simulink model "gm_HDLModulatorFull_vs"  (R2024a)
settings: Solver=FixedStepDiscrete  StartTime=0.0  StopTime=stopTime  RelTol=1e-3
values from neighbouring files (symbols this model uses):
  dataSymbols = [ ... (first row only)    [testModulatorFull.m]
undefined symbols (not defined in the file or in its folder): clk, clk_enable, fPHY, fs, interpolatorDelay, interpolatorFilter, N, numDataCarriers, oversamplingFactor, reset_x
libraries: hdlmdlgenlib x54, hdlsllib x21, dspsrcs4 x4, commdigbbndam3 x4, simulink x3, dspsigops x2, whdlutilities x1, dsphdlsigops2 x1, dsphdlfiltering2 x1, whdlmod x1, vivadosimlib x1, HDL_ieee_8021513 x1
settings Model: Creator=cotti  LastModifiedBy=cotti
settings OptimizationCC: BlockReduction=off  ConditionallyExecuteInputs=off  DefaultParameterBehavior=Inlined  InheritOutputTypeSmallerThanSingle=on
settings DebuggingCC: AlgebraicLoopMsg=error  ArtificialAlgebraicLoopMsg=error  InheritedTsInSrcMsg=none  SingleTaskRateTransMsg=error  UnconnectedInputMsg=warning  UnconnectedOutputMsg=warning  UnconnectedLineMsg=warning
settings HardwareCC: ProdBitPerPointer=32  ProdBitPerSizeT=32  ProdBitPerPtrDiffT=32  ProdLargestAtomicFloat=None  ProdIntDivRoundTo=Undefined  ProdEndianess=Unspecified  ProdWordSize=32  ProdHWDeviceType=ASIC/FPGA->ASIC/FPGA  TargetBitPerLong=64  TargetBitPerPointer=64  TargetBitPerSizeT=64  TargetBitPerPtrDiffT=64  TargetLongLongMode=on  TargetIntDivRoundTo=Zero  TargetEndianess=LittleEndian  TargetWordSize=64  TargetHWDeviceType=Custom Processor->MATLAB Host Computer  ProdEqTarget=off

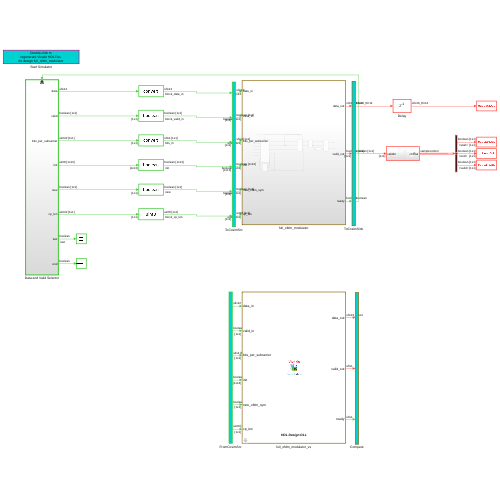
[thumbnail: Simulink's stored preview of the top-level diagram]
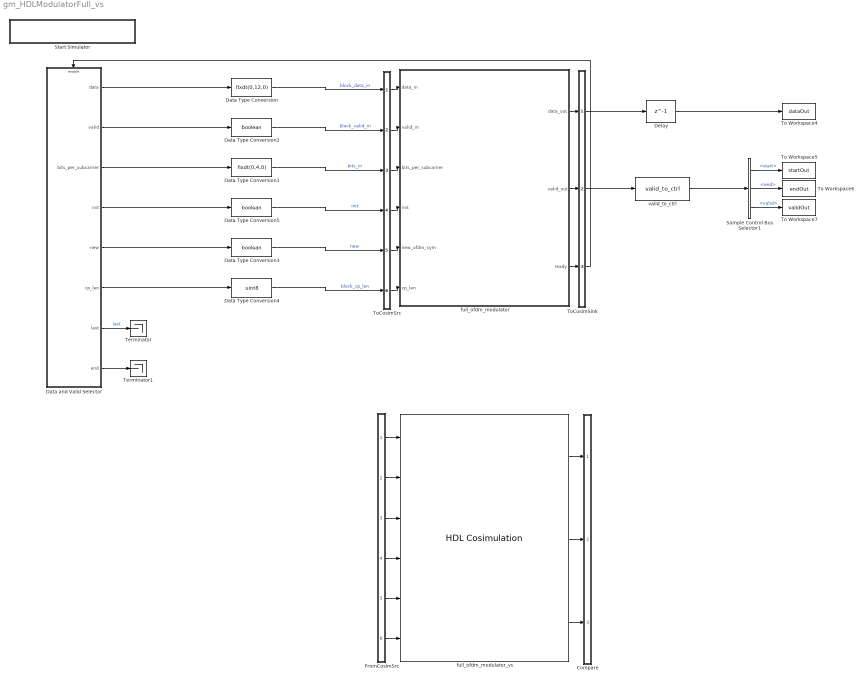
== system gm_HDLModulatorFull_vs ==
  Compare : Subsystem
      mask Display: disp('')
  Data Type Conversion : DataTypeConversion  OutDataTypeStr=fixdt(0,12,0)  SaturateOnIntegerOverflow=off  RndMeth=Floor  LockScale=on
  Data Type Conversion1 : DataTypeConversion  OutDataTypeStr=fixdt(0,4,0)  SaturateOnIntegerOverflow=off  RndMeth=Floor  LockScale=on
  Data Type Conversion2 : DataTypeConversion  OutDataTypeStr=boolean  SaturateOnIntegerOverflow=off  RndMeth=Floor  LockScale=on
  Data Type Conversion3 : DataTypeConversion  OutDataTypeStr=boolean  SaturateOnIntegerOverflow=off  RndMeth=Floor  LockScale=on
  Data Type Conversion4 : DataTypeConversion  OutDataTypeStr=uint8  SaturateOnIntegerOverflow=off  RndMeth=Floor  LockScale=on
  Data Type Conversion5 : DataTypeConversion  OutDataTypeStr=boolean  SaturateOnIntegerOverflow=off  RndMeth=Floor  LockScale=on
  Data and Valid Selector : Subsystem  TreatAsAtomicUnit=on
  Delay : Delay  DelayLength=1  InitialCondition=0  UseCircularBuffer=on
  FromCosimSrc : Subsystem
      mask Display: disp('')
  Sample Control Bus Selector1 : whdlutilities/Sample Control Bus Selector  OutputSignals=start,end,valid
  Start Simulator : Subsystem
      settings: OpenFcn=|
      | cosimDirName = pwd;
      | cd 'hdl_prj/hdlsrc/HDLModulatorFull';
      | [s,r] = system('vivado -mode batch -source gm_HDLModulatorFull_vs.tcl','-echo');
      | cd (cosimDirName);
      | clear cosimDirName;
      | if s
      |    error('Failed to create Vivado HDL design DLL using script gm_HDLModulatorFull_vs.tcl.');
      | end
      mask Display: disp('Double-click to\nregenerate Vivado HDL DLL\nfor design full_ofdm_modulator')
  Terminator : Terminator
  Terminator1 : Terminator
  To Workspace4 : ToWorkspace  VariableName=dataOut  SampleTime=1/fs
      settings: Save2DSignal=2-D array (concatenate along first dimension)
  To Workspace5 : ToWorkspace  VariableName=startOut  SampleTime=1/fs
      settings: Save2DSignal=2-D array (concatenate along first dimension)
  To Workspace6 : ToWorkspace  VariableName=endOut  SampleTime=1/fs
      settings: Save2DSignal=2-D array (concatenate along first dimension)
  To Workspace7 : ToWorkspace  VariableName=validOut  SampleTime=1/fs
      settings: Save2DSignal=2-D array (concatenate along first dimension)
  ToCosimSink : Subsystem
      mask Display: disp('')
  ToCosimSrc : Subsystem
      mask Display: disp('')
  full_ofdm_modulator : Subsystem
  full_ofdm_modulator_vs : vivadosimlib/HDL Cosimulation  PortPaths=/full_ofdm_modulator/data_in;/full_ofdm_modulator/valid_in;/full_ofdm_modulator/bits_per_subcarrier;/full_ofdm_modulator/init;/full_ofdm_modulator/new_ofdm_sym;/full_ofdm_modulator/cp_len;/full_ofdm_modulator/data_out;/full_ofdm_modulator/valid_out;/full_ofdm_modulator/ready  PortModes=[1 1 1 1 1 1 2 2 2 ]  PortTimes=[-1 -1 -1 -1 -1 -1 1.0000000000000000209225608301284726753266340892878361046314239502e-08 1.0000000000000000209225608301284726753266340892878361046314239502e-08 2.0000000000000000418451216602569453506532681785756722092628479004e-08 ]  PortSigns=[-1 -1 -1 -1 -1 -1 1 0 0 ]  PortFracLengths=[0,0,0,0,0,0,14,0,0]  PortWordLengths=[-1,-1,-1,-1,-1,-1,16,1,1]  PortHDLWordSizes=[12,1,4,1,1,8,16,1,1]  CommLocal=on  CommSharedMemory=on  CommPortNumber=4449  CommShowInfo=on  ClockPaths=clk;clk_enable;reset_x;  ClockModes=[2 4 3]  ClockTimes=[1e-08 3.7e-08 2.7e-08]  TclPostSimCommand="puts \"done\""  TimingMode=ns  TimingScaleFactor=1000000000  idxCellArray={'UNUSED_VAR'}  CosimBypass=Full Simulation  AllowDirectFeedthrough=on  ProductName=EDA Simulator Link VS  RunAutoTimescale=off  HdlClocks=0  PreRunTime=40  PreRunTimeUnit=ns
  valid_to_ctrl : HDL_ieee_8021513/valid_to_ctrl  SystemSampleTime=-1  VariantActivationTime=update diagram  AllowFlexibleInterface=on  Latency=0  AutoFrameSizeCalculation=off
      settings: SourceProductName=HDL IEEE 8021513
  wires:
  Sample Control Bus Selector1/3 -> To Workspace7/1  "<valid>"
  valid_to_ctrl/1 -> Sample Control Bus Selector1/1
  Sample Control Bus Selector1/1 -> To Workspace5/1  "<start>"
  Sample Control Bus Selector1/2 -> To Workspace6/1  "<end>"
  Data and Valid Selector/8(end) -> Terminator1/1
  Data and Valid Selector/6(cp_len) -> Data Type Conversion4/1
  Data and Valid Selector/4(init) -> Data Type Conversion5/1
  Data and Valid Selector/2(valid) -> Data Type Conversion2/1
  Data and Valid Selector/1(data) -> Data Type Conversion/1
  Data and Valid Selector/3(bits_per_subcarrier) -> Data Type Conversion1/1
  Data and Valid Selector/5(new) -> Data Type Conversion3/1
  Data and Valid Selector/7(last) -> Terminator/1  "last"
  Delay/1 -> To Workspace4/1
  ToCosimSrc/1(out1) -> full_ofdm_modulator/1(data_in)
  ToCosimSrc/2(out2) -> full_ofdm_modulator/2(valid_in)
  ToCosimSrc/3(out3) -> full_ofdm_modulator/3(bits_per_subcarrier)
  ToCosimSrc/4(out4) -> full_ofdm_modulator/4(init)
  ToCosimSrc/5(out5) -> full_ofdm_modulator/5(new_ofdm_sym)
  ToCosimSrc/6(out6) -> full_ofdm_modulator/6(cp_len)
  full_ofdm_modulator/1(data_out) -> ToCosimSink/1(in1)
  full_ofdm_modulator/2(valid_out) -> ToCosimSink/2(in2)
  full_ofdm_modulator/3(ready) -> ToCosimSink/3(in3)
  Data Type Conversion/1 -> ToCosimSrc/1(in1)  "block_data_in"
  Data Type Conversion2/1 -> ToCosimSrc/2(in2)  "block_valid_in"
  Data Type Conversion1/1 -> ToCosimSrc/3(in3)  "bits_in"
  Data Type Conversion5/1 -> ToCosimSrc/4(in4)  "init"
  Data Type Conversion3/1 -> ToCosimSrc/5(in5)  "new"
  Data Type Conversion4/1 -> ToCosimSrc/6(in6)  "block_cp_len"
  ToCosimSink/1(out1) -> Delay/1
  ToCosimSink/2(out2) -> valid_to_ctrl/1
  ToCosimSink/3(out3) -> Data and Valid Selector/Enable
  FromCosimSrc/1(out1) -> full_ofdm_modulator_vs/1
  FromCosimSrc/2(out2) -> full_ofdm_modulator_vs/2
  FromCosimSrc/3(out3) -> full_ofdm_modulator_vs/3
  FromCosimSrc/4(out4) -> full_ofdm_modulator_vs/4
  FromCosimSrc/5(out5) -> full_ofdm_modulator_vs/5
  FromCosimSrc/6(out6) -> full_ofdm_modulator_vs/6
  full_ofdm_modulator_vs/1 -> Compare/1(in1)
  full_ofdm_modulator_vs/2 -> Compare/2(in2)
  full_ofdm_modulator_vs/3 -> Compare/3(in3)

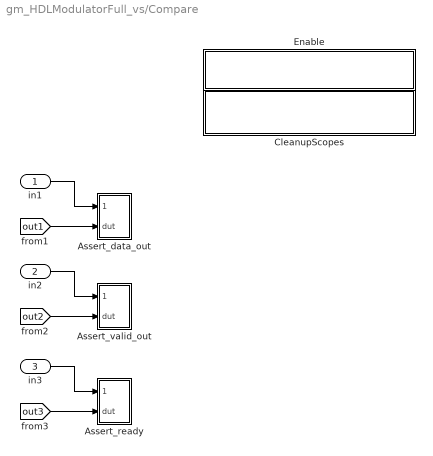
== system gm_HDLModulatorFull_vs/Compare ==
  in1 : Inport
  in2 : Inport  Port=2
  in3 : Inport  Port=3
  Assert_data_out : Subsystem
      settings: LibrarySourceBlock=hdlmdlgenlib/AssertEq
  Assert_ready : Subsystem
      settings: LibrarySourceBlock=hdlmdlgenlib/AssertEq
  Assert_valid_out : Subsystem
      settings: LibrarySourceBlock=hdlmdlgenlib/AssertEq
  CleanupScopes : Subsystem
      settings: OpenFcn=|
      | blkName = gcb; %self block
      | idx = regexp(blkName, '/CleanupScopes$', 'once');
      | blkParent = blkName(1:idx-1);
      | blks=find_system(blkParent, 'LookUnderMasks', 'all','blocktype', 'Scope');
      | for itr = 1:length(blks)
      | 	 hScopeCfg = get_param(blks{itr},'ScopeConfiguration');
      | 	 hScopeCfg.Visible = ~ hScopeCfg.Visible;
      | end
      | drawnow;
      mask Display: fprintf(message('hdlcoder:cosim:vnl_dblclick').getString());
  Enable : Subsystem
      settings: OpenFcn=|
      | blkName = gcb;
      | idx = regexp(blkName, '/Enable$', 'once');
      | blkParent = blkName(1:idx-1);
      | blks=find_system(blkParent, 'LookUnderMasks', 'all','blocktype', 'Assertion');
      | e = get_param(blks{1}, 'Enabled');
      | if strcmp(e, 'on'), f= 'off';, else, f = 'on';, end
      | for ii=1:length(blks), set_param(blks{ii}, 'Enabled', f);, end
      | set_param(gcb, 'MaskDisplay',['fprintf(message(''hdlcoder:cosim:vnl_dblclick_assertions'',','''',upper(e),'''',').getString())']);
      mask Display: fprintf(message('hdlcoder:cosim:vnl_dblclick_assertions','OFF').getString());
  wires:
  in3/1 -> Assert_ready/1(cosim)
  [out2] -> Assert_valid_out/2(dut)
  [out3] -> Assert_ready/2(dut)
  in2/1 -> Assert_valid_out/1(cosim)
  [out1] -> Assert_data_out/2(dut)
  in1/1 -> Assert_data_out/1(cosim)

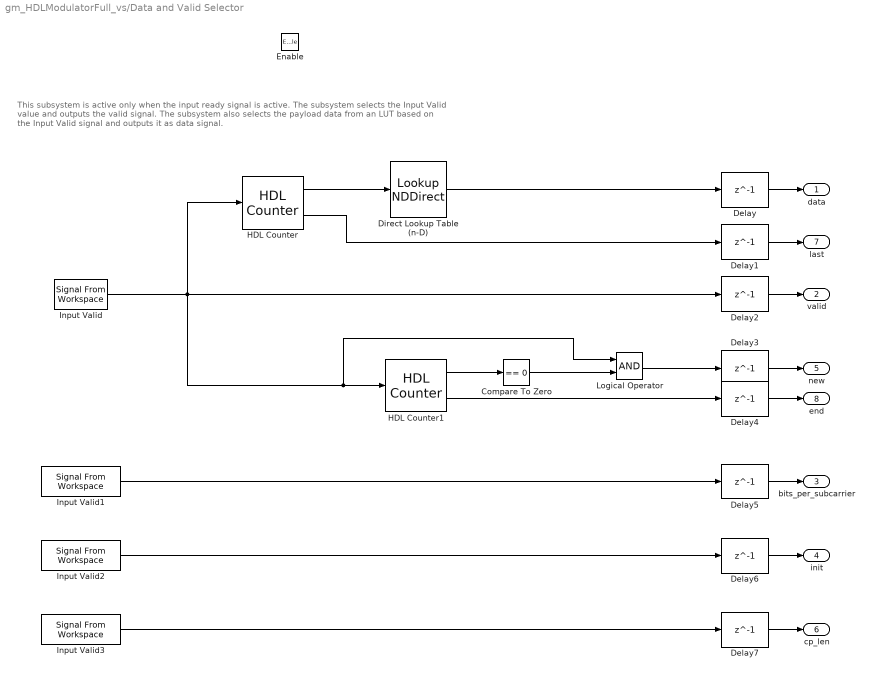
== system gm_HDLModulatorFull_vs/Data and Valid Selector ==
  note: This subsystem is active only when the input ready signal is active. The subsystem selects the Input Valid value and outputs the valid signal.
      | The subsystem also selects the payload data from an LUT based on the Input Valid signal and outputs it as data signal.
  Enable : EnablePort
  Compare To Zero : hdlsllib/Logic and Bit Operations/Compare To Zero  relop===  OutDataTypeStr=boolean
  Delay{,1..7} (8 alike) : Delay  DelayLength=1  InitialCondition=0  UseCircularBuffer=on
  Direct Lookup Table (n-D) : LookupNDDirect  NumberOfTableDimensions=1  Table=dataSymbols  DiagnosticForOutOfRangeInput=Error  TableDataTypeStr=fixdt(0,12,0)
  HDL Counter : hdlsllib/Sources/HDL Counter  CountType=Count limited  CountInit=0  CountStep=1  CountMax=length(dataSymbols) -1  CountFromType=Initial value  CountFrom=0  CountResetPort=off  CountLoadPort=off  CountEnbPort=on  CountDirPort=off  CountHitOutputPort=on  CountDataType=Unsigned  CountWordLen=nextpow2(length(dataSymbols))  CountFracLen=0  CountSampTime=1
  HDL Counter1 : hdlsllib/Sources/HDL Counter  CountType=Count limited  CountInit=0  CountStep=1  CountMax=numDataCarriers-1  CountFromType=Initial value  CountFrom=0  CountResetPort=off  CountLoadPort=off  CountEnbPort=on  CountDirPort=off  CountHitOutputPort=on  CountDataType=Unsigned  CountWordLen=nextpow2(numDataCarriers)  CountFracLen=0  CountSampTime=1
  Input Valid : dspsrcs4/Signal From Workspace  X=validIn  Ts=1/fPHY  nsamps=1  OutputAfterFinalValue=Setting to zero  ignoreOrWarnInputAndFrameLengths=off  OutputFrames=off
  Input Valid1 : dspsrcs4/Signal From Workspace  X=bitsPerSubcarrier  Ts=1/fPHY  nsamps=1  OutputAfterFinalValue=Setting to zero  ignoreOrWarnInputAndFrameLengths=off  OutputFrames=off
  Input Valid2 : dspsrcs4/Signal From Workspace  X=init  Ts=1/fPHY  nsamps=1  OutputAfterFinalValue=Setting to zero  ignoreOrWarnInputAndFrameLengths=off  OutputFrames=off
  Input Valid3 : dspsrcs4/Signal From Workspace  X=cpLen  Ts=1/fPHY  nsamps=1  OutputAfterFinalValue=Setting to zero  ignoreOrWarnInputAndFrameLengths=off  OutputFrames=off
  Logical Operator : Logic  AllPortsSameDT=off  OutDataTypeStr=boolean
  data : Outport  InitialOutput=0  VectorParamsAs1DForOutWhenUnconnected=off
  valid : Outport  Port=2  InitialOutput=0  VectorParamsAs1DForOutWhenUnconnected=off
  bits_per_subcarrier : Outport  Port=3  VectorParamsAs1DForOutWhenUnconnected=off
  init : Outport  Port=4  VectorParamsAs1DForOutWhenUnconnected=off
  new : Outport  Port=5  VectorParamsAs1DForOutWhenUnconnected=off
  cp_len : Outport  Port=6  VectorParamsAs1DForOutWhenUnconnected=off
  last : Outport  Port=7  VectorParamsAs1DForOutWhenUnconnected=off
  end : Outport  Port=8  VectorParamsAs1DForOutWhenUnconnected=off
  wires:
  HDL Counter/1 -> Direct Lookup Table (n-D)/1
  Direct Lookup Table (n-D)/1 -> Delay/1
  HDL Counter/2 -> Delay1/1
  HDL Counter1/1 -> Compare To Zero/1
  Compare To Zero/1 -> Logical Operator/2
  Logical Operator/1 -> Delay3/1
  HDL Counter1/2 -> Delay4/1
  Input Valid/1 -> HDL Counter/1, Delay2/1, Logical Operator/1, HDL Counter1/1
  Input Valid3/1 -> Delay7/1
  Input Valid2/1 -> Delay6/1
  Input Valid1/1 -> Delay5/1
  Delay/1 -> data/1
  Delay1/1 -> last/1
  Delay2/1 -> valid/1
  Delay3/1 -> new/1
  Delay4/1 -> end/1
  Delay5/1 -> bits_per_subcarrier/1
  Delay6/1 -> init/1
  Delay7/1 -> cp_len/1

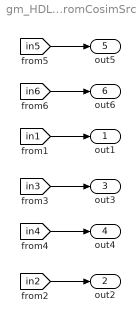
== system gm_HDLModulatorFull_vs/FromCosimSrc ==
  out1 : Outport
  out2 : Outport  Port=2
  out3 : Outport  Port=3
  out4 : Outport  Port=4
  out5 : Outport  Port=5
  out6 : Outport  Port=6
  wires:
  [in2] -> out2/1
  [in3] -> out3/1
  [in6] -> out6/1
  [in4] -> out4/1
  [in1] -> out1/1
  [in5] -> out5/1

== system gm_HDLModulatorFull_vs/Start Simulator ==

== system gm_HDLModulatorFull_vs/ToCosimSink ==
  in1 : Inport
  in2 : Inport  Port=2
  in3 : Inport  Port=3
  out1 : Outport
  out2 : Outport  Port=2
  out3 : Outport  Port=3
  tag scope: out1=global, out2=global, out3=global
  wires:
  in1/1 -> out1/1, [out1]
  in2/1 -> out2/1, [out2]
  in3/1 -> out3/1, [out3]

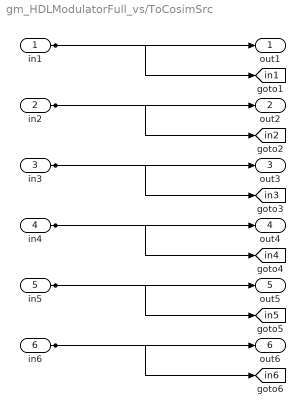
== system gm_HDLModulatorFull_vs/ToCosimSrc ==
  in1 : Inport
  in2 : Inport  Port=2
  in3 : Inport  Port=3
  in4 : Inport  Port=4
  in5 : Inport  Port=5
  in6 : Inport  Port=6
  out1 : Outport
  out2 : Outport  Port=2
  out3 : Outport  Port=3
  out4 : Outport  Port=4
  out5 : Outport  Port=5
  out6 : Outport  Port=6
  tag scope: in1=global, in2=global, in3=global, in4=global, in5=global, in6=global
  wires:
  in1/1 -> out1/1, [in1]
  in2/1 -> out2/1, [in2]
  in3/1 -> out3/1, [in3]
  in4/1 -> out4/1, [in4]
  in5/1 -> out5/1, [in5]
  in6/1 -> out6/1, [in6]

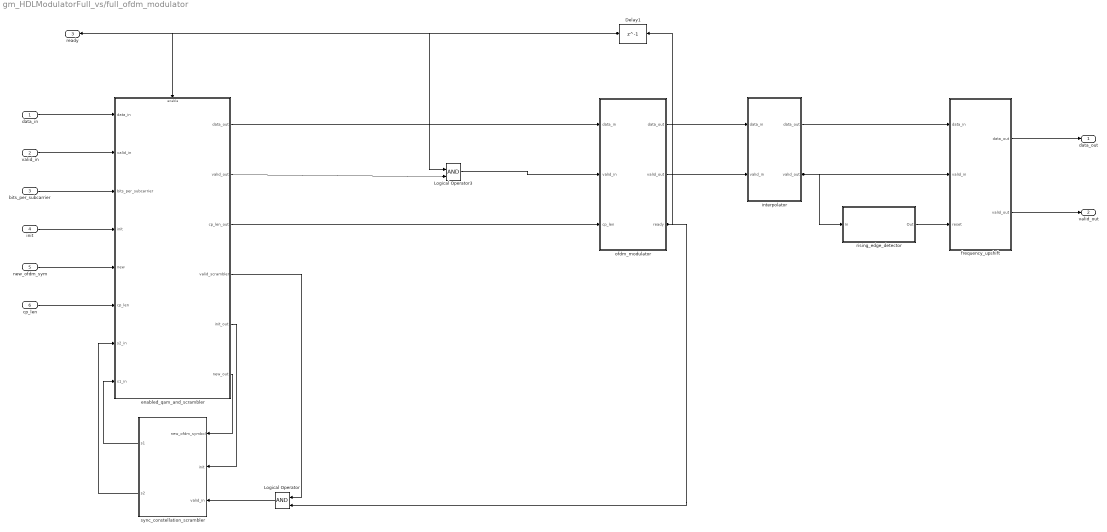
== system gm_HDLModulatorFull_vs/full_ofdm_modulator ==
  data_in : Inport  OutDataTypeStr=fixdt(0, 12, 0)  SampleTime=2e-08
  valid_in : Inport  Port=2  OutDataTypeStr=boolean  SampleTime=2e-08
  bits_per_subcarrier : Inport  Port=3  OutDataTypeStr=fixdt(0, 4, 0)  SampleTime=2e-08
  init : Inport  Port=4  OutDataTypeStr=boolean  PortDimensions=[1 13]  SampleTime=2e-08
  new_ofdm_sym : Inport  Port=5  OutDataTypeStr=boolean  SampleTime=2e-08
  cp_len : Inport  Port=6  OutDataTypeStr=uint8  SampleTime=2e-08
  Delay1 : Delay  DelayLength=1  InitialCondition=0  UseCircularBuffer=on
  Logical Operator : Logic  IconShape=distinctive  AllPortsSameDT=off  OutDataTypeStr=boolean
  Logical Operator3 : Logic  IconShape=distinctive  AllPortsSameDT=off  OutDataTypeStr=boolean
  enabled_qam_and_scrambler : Subsystem
  frequency_upshift : Subsystem
  interpolator : Subsystem
  ofdm_modulator : Subsystem
  rising_edge_detector : Subsystem
  sync_constellation_scrambler : Subsystem
  data_out : Outport  SampleTime=1e-08
  valid_out : Outport  Port=2  SampleTime=1e-08
  ready : Outport  Port=3  SampleTime=2e-08
  wires:
  sync_constellation_scrambler/2(s2) -> enabled_qam_and_scrambler/7(s2_in)
  sync_constellation_scrambler/1(s1) -> enabled_qam_and_scrambler/8(s1_in)
  rising_edge_detector/1(Out) -> frequency_upshift/3(reset)
  ofdm_modulator/3(ready) -> Delay1/1, Logical Operator/2
  ofdm_modulator/2(valid_out) -> interpolator/2(valid_in)
  ofdm_modulator/1(data_out) -> interpolator/1(data_in)
  interpolator/2(valid_out) -> rising_edge_detector/1(In), frequency_upshift/2(valid_in)
  interpolator/1(data_out) -> frequency_upshift/1(data_in)
  frequency_upshift/2(valid_out) -> valid_out/1
  frequency_upshift/1(data_out) -> data_out/1
  enabled_qam_and_scrambler/6(new_out) -> sync_constellation_scrambler/1(new_ofdm_symbol)
  enabled_qam_and_scrambler/5(init_out) -> sync_constellation_scrambler/2(init)
  enabled_qam_and_scrambler/4(valid_scrambler) -> Logical Operator/1
  enabled_qam_and_scrambler/3(cp_len_out) -> ofdm_modulator/3(cp_len)
  enabled_qam_and_scrambler/2(valid_out) -> Logical Operator3/2
  enabled_qam_and_scrambler/1(data_out) -> ofdm_modulator/1(data_in)
  Logical Operator3/1 -> ofdm_modulator/2(valid_in)
  Logical Operator/1 -> sync_constellation_scrambler/3(valid_in)
  Delay1/1 -> enabled_qam_and_scrambler/Enable, ready/1, Logical Operator3/1
  cp_len/1 -> enabled_qam_and_scrambler/6(cp_len)
  new_ofdm_sym/1 -> enabled_qam_and_scrambler/5(new)
  init/1 -> enabled_qam_and_scrambler/4(init)
  bits_per_subcarrier/1 -> enabled_qam_and_scrambler/3(bits_per_subcarrier)
  valid_in/1 -> enabled_qam_and_scrambler/2(valid_in)
  data_in/1 -> enabled_qam_and_scrambler/1(data_in)

== system gm_HDLModulatorFull_vs/Compare/Assert_data_out ==
  cosim : Inport
  dut : Inport  Port=2
  AssertEq : Assertion
  Compare To Zero : simulink/Logic and Bit Operations/Compare To Zero  relop===  OutDataTypeStr=boolean
  Relational Operator : RelationalOperator  Operator===  OutDataTypeStr=boolean  InputSameDT=off
  compare: data_out : Scope  NumInputPorts=3
  wires:
  Compare To Zero/1 -> compare: data_out/3  "err"
  Relational Operator/1 -> Compare To Zero/1, AssertEq/1
  cosim/1 -> compare: data_out/1, Relational Operator/1  "cosim"
  dut/1 -> compare: data_out/2, Relational Operator/2  "dut ref"

== system gm_HDLModulatorFull_vs/Compare/Assert_ready ==
  cosim : Inport
  dut : Inport  Port=2
  AssertEq : Assertion
  Compare To Zero : simulink/Logic and Bit Operations/Compare To Zero  relop===  OutDataTypeStr=boolean
  Relational Operator : RelationalOperator  Operator===  OutDataTypeStr=boolean  InputSameDT=off
  compare: ready : Scope  NumInputPorts=3
  wires:
  Compare To Zero/1 -> compare: ready/3  "err"
  Relational Operator/1 -> Compare To Zero/1, AssertEq/1
  cosim/1 -> compare: ready/1, Relational Operator/1  "cosim"
  dut/1 -> compare: ready/2, Relational Operator/2  "dut ref"

== system gm_HDLModulatorFull_vs/Compare/Assert_valid_out ==
  cosim : Inport
  dut : Inport  Port=2
  AssertEq : Assertion
  Compare To Zero : simulink/Logic and Bit Operations/Compare To Zero  relop===  OutDataTypeStr=boolean
  Relational Operator : RelationalOperator  Operator===  OutDataTypeStr=boolean  InputSameDT=off
  compare: valid_out : Scope  NumInputPorts=3
  wires:
  Compare To Zero/1 -> compare: valid_out/3  "err"
  Relational Operator/1 -> Compare To Zero/1, AssertEq/1
  cosim/1 -> compare: valid_out/1, Relational Operator/1  "cosim"
  dut/1 -> compare: valid_out/2, Relational Operator/2  "dut ref"

== system gm_HDLModulatorFull_vs/Compare/CleanupScopes ==

== system gm_HDLModulatorFull_vs/Compare/Enable ==

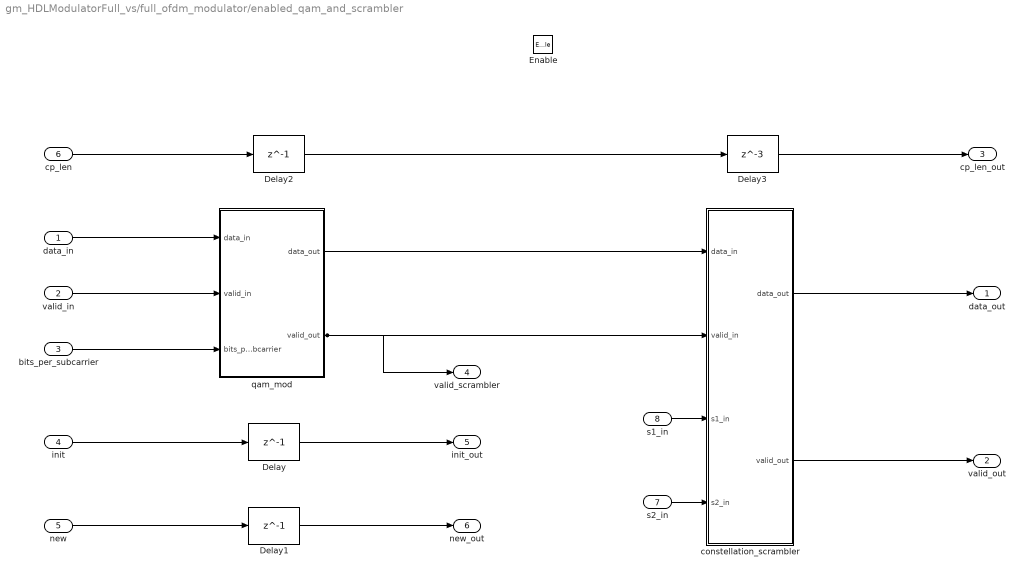
== system gm_HDLModulatorFull_vs/full_ofdm_modulator/enabled_qam_and_scrambler ==
  data_in : Inport  OutDataTypeStr=fixdt(0, 12, 0)  PortDimensions=1  SampleTime=2e-08
  valid_in : Inport  Port=2  OutDataTypeStr=boolean  PortDimensions=1  SampleTime=2e-08
  bits_per_subcarrier : Inport  Port=3  OutDataTypeStr=fixdt(0, 4, 0)  PortDimensions=1  SampleTime=2e-08
  init : Inport  Port=4  OutDataTypeStr=boolean  PortDimensions=[1 13]  SampleTime=2e-08
  new : Inport  Port=5  OutDataTypeStr=boolean  PortDimensions=1  SampleTime=2e-08
  cp_len : Inport  Port=6  OutDataTypeStr=uint8  PortDimensions=1  SampleTime=2e-08
  s2_in : Inport  Port=7  OutDataTypeStr=boolean  PortDimensions=1  SampleTime=2e-08
  s1_in : Inport  Port=8  OutDataTypeStr=boolean  PortDimensions=1  SampleTime=2e-08
  Enable : EnablePort  OutDataTypeStr=boolean
  Delay : Delay  DelayLength=1  InitialCondition=0  UseCircularBuffer=on
  Delay1 : Delay  DelayLength=1  InitialCondition=0  UseCircularBuffer=on
  Delay2 : Delay  DelayLength=1  InitialCondition=0  UseCircularBuffer=on
  Delay3 : Delay  DelayLength=3  InitialCondition=0  UseCircularBuffer=on
  constellation_scrambler : Subsystem
  qam_mod : Subsystem
  data_out : Outport  SampleTime=2e-08  InitialOutput=0  VectorParamsAs1DForOutWhenUnconnected=off
  valid_out : Outport  Port=2  SampleTime=2e-08  InitialOutput=0  VectorParamsAs1DForOutWhenUnconnected=off
  cp_len_out : Outport  Port=3  SampleTime=2e-08  InitialOutput=0  VectorParamsAs1DForOutWhenUnconnected=off
  valid_scrambler : Outport  Port=4  SampleTime=2e-08  InitialOutput=0  VectorParamsAs1DForOutWhenUnconnected=off
  init_out : Outport  Port=5  SampleTime=2e-08  InitialOutput=0  VectorParamsAs1DForOutWhenUnconnected=off
  new_out : Outport  Port=6  SampleTime=2e-08  InitialOutput=0  VectorParamsAs1DForOutWhenUnconnected=off
  wires:
  qam_mod/2(valid_out) -> constellation_scrambler/2(valid_in), valid_scrambler/1
  qam_mod/1(data_out) -> constellation_scrambler/1(data_in)
  constellation_scrambler/2(valid_out) -> valid_out/1
  constellation_scrambler/1(data_out) -> data_out/1
  Delay3/1 -> cp_len_out/1
  Delay2/1 -> Delay3/1
  Delay1/1 -> new_out/1
  Delay/1 -> init_out/1
  s1_in/1 -> constellation_scrambler/3(s1_in)
  s2_in/1 -> constellation_scrambler/4(s2_in)
  cp_len/1 -> Delay2/1
  new/1 -> Delay1/1
  init/1 -> Delay/1
  bits_per_subcarrier/1 -> qam_mod/3(bits_per_subcarrier)
  valid_in/1 -> qam_mod/2(valid_in)
  data_in/1 -> qam_mod/1(data_in)

== system gm_HDLModulatorFull_vs/full_ofdm_modulator/frequency_upshift ==
  data_in : Inport  OutDataTypeStr=fixdt(1, 16, 14)  SampleTime=1e-08
      settings: SignalType=complex
  valid_in : Inport  Port=2  OutDataTypeStr=boolean  SampleTime=1e-08
  reset : Inport  Port=3  OutDataTypeStr=boolean  SampleTime=1e-08
  Delay : Delay  DelayLength=6  InitialCondition=0  UseCircularBuffer=on
  Delay1 : Delay  DelayLength=4  InitialCondition=0  UseCircularBuffer=on
  Delay2 : Delay  DelayLength=1  InitialCondition=0  UseCircularBuffer=on
  Delay3 : Delay  DelayLength=1  InitialCondition=0  UseCircularBuffer=on
  Mixer : Subsystem
  NCO : dsphdlsigops2/NCO  PhaseIncrementSource=Property  PhaseIncrement=ncoPhaseIncrement  PhaseOffsetSource=Property  PhaseOffset=0  DitherSource=None  NumDitherBits=1  SamplesPerFrame=1  LUTCompress=off  ResetAction=on  Waveform=Complex exponential  PhasePort=off  SimulateUsing=Code generation  AccumulatorWL=ncoWordLength  PhaseQuantization=off  NumQuantizerAccumulatorBits=6  OutputDataType=Binary point scaling  OutputWL=16  OutputFL=14
  data_out : Outport  SampleTime=1e-08
  valid_out : Outport  Port=2  SampleTime=1e-08
  wires:
  NCO/2 -> Delay1/1
  NCO/1 -> Mixer/2(ncoIn)
  Mixer/1(mixedOut) -> data_out/1
  Delay3/1 -> Delay/1
  Delay2/1 -> NCO/2
  Delay1/1 -> valid_out/1
  Delay/1 -> Mixer/1(dataIn)
  reset/1 -> NCO/1
  valid_in/1 -> Delay2/1
  data_in/1 -> Delay3/1

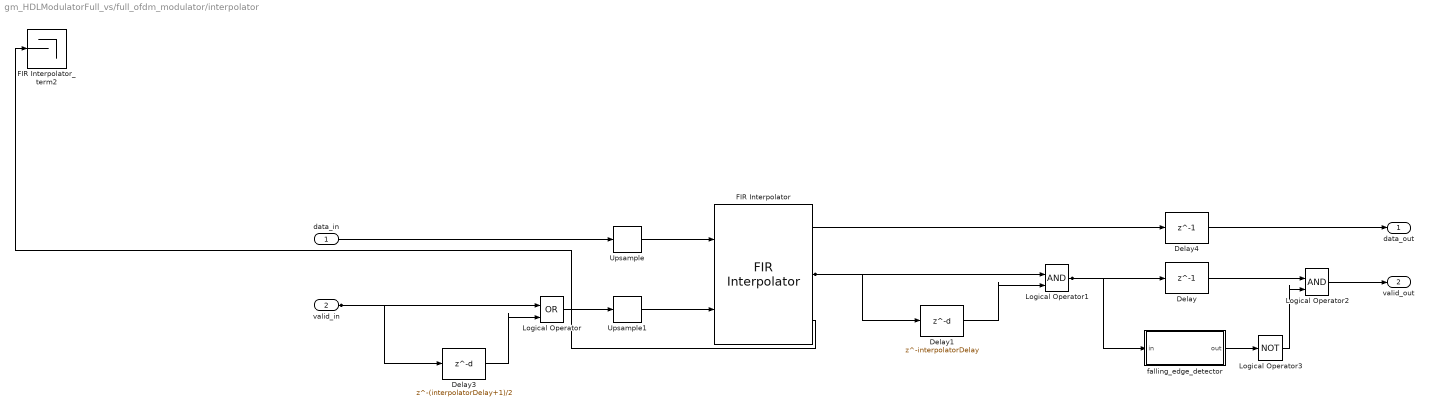
== system gm_HDLModulatorFull_vs/full_ofdm_modulator/interpolator ==
  data_in : Inport  OutDataTypeStr=fixdt(1, 16, 14)  SampleTime=2e-08
      settings: SignalType=complex
  valid_in : Inport  Port=2  OutDataTypeStr=boolean  SampleTime=2e-08
  Delay : Delay  DelayLength=1  InitialCondition=0  UseCircularBuffer=on
  Delay1 : Delay  DelayLength=interpolatorDelay  InitialCondition=0  UseCircularBuffer=on
  Delay3 : Delay  DelayLength=(interpolatorDelay+1)/2  InitialCondition=0  UseCircularBuffer=on
  Delay4 : Delay  DelayLength=1  InitialCondition=0  UseCircularBuffer=on
  FIR Interpolator : dsphdlfiltering2/FIR Interpolator  Numerator=interpolatorFilter.Numerator  FilterStructure=Direct form systolic  InterpolationFactor=oversamplingFactor  NumCycles=oversamplingFactor  SimulateUsing=Code generation  roundingMode=Floor  overflowMode=off  CoefficientsDataTypeStr=fixdt(1,16,14)  OutputDataTypeStr=fixdt(1,16,14)  ResetInputPort=off  HDLGlobalReset=off
  FIR Interpolator_term2 : Terminator
  Logical Operator : Logic  Operator=OR  IconShape=distinctive  AllPortsSameDT=off  OutDataTypeStr=boolean
  Logical Operator1 : Logic  IconShape=distinctive  AllPortsSameDT=off  OutDataTypeStr=boolean
  Logical Operator2 : Logic  IconShape=distinctive  AllPortsSameDT=off  OutDataTypeStr=boolean
  Logical Operator3 : Logic  Operator=NOT  IconShape=distinctive  AllPortsSameDT=off  OutDataTypeStr=boolean
  Upsample : dspsigops/Upsample  FactorSource=Dialog parameter  N=oversamplingFactor  Nmax=16  phase=0  RateOptions=Allow multirate processing  ic=0  mode=Unused parameter value
      settings: LibrarySourceBlock=dsphdlsupportsigops/Upsample
  Upsample1 : dspsigops/Upsample  FactorSource=Dialog parameter  N=oversamplingFactor  Nmax=16  phase=0  RateOptions=Allow multirate processing  ic=0  mode=Unused parameter value
      settings: LibrarySourceBlock=dsphdlsupportsigops/Upsample
  falling_edge_detector : Subsystem
  data_out : Outport  SampleTime=1e-08
  valid_out : Outport  Port=2  SampleTime=1e-08
  wires:
  falling_edge_detector/1(out) -> Logical Operator3/1
  Upsample1/1 -> FIR Interpolator/2
  Upsample/1 -> FIR Interpolator/1
  Logical Operator3/1 -> Logical Operator2/2
  Logical Operator2/1 -> valid_out/1
  Logical Operator1/1 -> falling_edge_detector/1(in), Delay/1
  Logical Operator/1 -> Upsample1/1
  FIR Interpolator/3 -> FIR Interpolator_term2/1
  FIR Interpolator/2 -> Delay1/1, Logical Operator1/1
  FIR Interpolator/1 -> Delay4/1
  Delay4/1 -> data_out/1
  Delay3/1 -> Logical Operator/2
  Delay1/1 -> Logical Operator1/2
  Delay/1 -> Logical Operator2/1
  valid_in/1 -> Delay3/1, Logical Operator/1
  data_in/1 -> Upsample/1

== system gm_HDLModulatorFull_vs/full_ofdm_modulator/ofdm_modulator ==
  data_in : Inport  OutDataTypeStr=fixdt(1, 16, 14)  SampleTime=2e-08
      settings: SignalType=complex
  valid_in : Inport  Port=2  OutDataTypeStr=boolean  SampleTime=2e-08
  cp_len : Inport  Port=3  OutDataTypeStr=uint8  SampleTime=2e-08
  Constant2 : Constant  Value=N  OutDataTypeStr=fixdt(0,9,0)  SampleTime=-1  LockScale=on
  Constant3 : Constant  Value=0  OutDataTypeStr=fixdt(0,2,0)  SampleTime=-1  LockScale=on
  Constant4 : Constant  Value=11  OutDataTypeStr=fixdt(0,4,0)  SampleTime=-1  LockScale=on
  OFDM Modulator : whdlmod/OFDM Modulator  OFDMParametersSource=Input Port  FFTLength=64  MaxFFTLength=N  CPLength=16  numLgSc=6  numRgSc=5  InsertDCNull=off  Windowing=off  WindowLength=4  MaxWindowLength=8  ResetInputPort=off  Normalize=on  RoundingMethod=Floor  SimulateUsing=Code generation
  data_out : Outport  SampleTime=2e-08
  valid_out : Outport  Port=2  SampleTime=2e-08
  ready : Outport  Port=3  SampleTime=2e-08
  wires:
  OFDM Modulator/3 -> ready/1
  OFDM Modulator/2 -> valid_out/1
  OFDM Modulator/1 -> data_out/1
  Constant4/1 -> OFDM Modulator/5
  Constant3/1 -> OFDM Modulator/6
  Constant2/1 -> OFDM Modulator/3
  cp_len/1 -> OFDM Modulator/4
  valid_in/1 -> OFDM Modulator/2
  data_in/1 -> OFDM Modulator/1

== system gm_HDLModulatorFull_vs/full_ofdm_modulator/rising_edge_detector ==
  In : Inport  OutDataTypeStr=boolean  SampleTime=1e-08
  Delay2 : Delay  DelayLength=1  InitialCondition=0  UseCircularBuffer=on
  Logical Operator1 : Logic  IconShape=distinctive  AllPortsSameDT=off  OutDataTypeStr=boolean
  Logical Operator2 : Logic  Operator=NOT  IconShape=distinctive  AllPortsSameDT=off  OutDataTypeStr=boolean
  Out : Outport  SampleTime=1e-08
  wires:
  Logical Operator2/1 -> Logical Operator1/2
  Logical Operator1/1 -> Out/1
  Delay2/1 -> Logical Operator2/1
  In/1 -> Delay2/1, Logical Operator1/1

== system gm_HDLModulatorFull_vs/full_ofdm_modulator/sync_constellation_scrambler ==
  new_ofdm_symbol : Inport  OutDataTypeStr=boolean  SampleTime=2e-08
  init : Inport  Port=2  OutDataTypeStr=boolean  PortDimensions=[1 13]  SampleTime=2e-08
  valid_in : Inport  Port=3  OutDataTypeStr=boolean  SampleTime=2e-08
  Rate Transition : RateTransition  OutPortSampleTime=1/fPHY
  Rate Transition1 : RateTransition  OutPortSampleTime=1/fPHY
  Rate Transition2 : RateTransition  OutPortSampleTime=1/(2*fPHY)
  Rate Transition3 : RateTransition  OutPortSampleTime=1/(2*fPHY)
  Rate Transition4 : RateTransition  OutPortSampleTime=1/(2*fPHY)
  Synchronous constellation scrambler : Subsystem
  s1 : Outport  SampleTime=2e-08
  s2 : Outport  Port=2  SampleTime=2e-08
  wires:
  Synchronous constellation scrambler/2(s2_out) -> Rate Transition/1
  Synchronous constellation scrambler/1(s1_out) -> Rate Transition1/1
  Rate Transition4/1 -> Synchronous constellation scrambler/1(valid_in)
  Rate Transition3/1 -> Synchronous constellation scrambler/2(init)
  Rate Transition2/1 -> Synchronous constellation scrambler/3(new_ofdm_symbol)
  Rate Transition1/1 -> s1/1
  Rate Transition/1 -> s2/1
  valid_in/1 -> Rate Transition4/1
  init/1 -> Rate Transition3/1
  new_ofdm_symbol/1 -> Rate Transition2/1

== system gm_HDLModulatorFull_vs/full_ofdm_modulator/enabled_qam_and_scrambler/constellation_scrambler ==
  data_in : Inport  OutDataTypeStr=fixdt(1, 16, 14)  SampleTime=2e-08
      settings: SignalType=complex
  valid_in : Inport  Port=2  OutDataTypeStr=boolean  SampleTime=2e-08
  s1_in : Inport  Port=3  OutDataTypeStr=boolean  SampleTime=2e-08
  s2_in : Inport  Port=4  OutDataTypeStr=boolean  SampleTime=2e-08
  Delay : Delay  InitialCondition=0  UseCircularBuffer=on
  Delay1 : Delay  InitialCondition=0  UseCircularBuffer=on
  Delay2 : Delay  DelayLength=1  InitialCondition=0  UseCircularBuffer=on
  Delay3 : Delay  DelayLength=1  InitialCondition=0  UseCircularBuffer=on
  rotate : Subsystem
  data_out : Outport  SampleTime=2e-08  InitialOutput=0
  valid_out : Outport  Port=2  SampleTime=2e-08  InitialOutput=0
  wires:
  rotate/1(data_out) -> Delay2/1
  Delay3/1 -> valid_out/1
  Delay2/1 -> data_out/1
  Delay1/1 -> Delay3/1
  Delay/1 -> rotate/3(data_in)
  s2_in/1 -> rotate/1(s2)
  s1_in/1 -> rotate/2(s1)
  valid_in/1 -> Delay1/1
  data_in/1 -> Delay/1

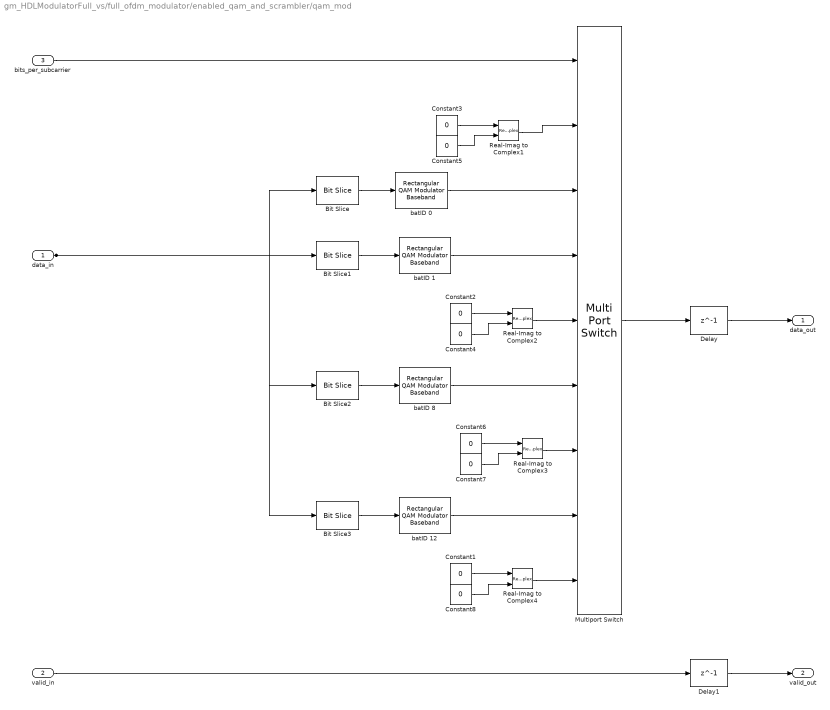
== system gm_HDLModulatorFull_vs/full_ofdm_modulator/enabled_qam_and_scrambler/qam_mod ==
  data_in : Inport  OutDataTypeStr=fixdt(0, 12, 0)  SampleTime=2e-08
  valid_in : Inport  Port=2  OutDataTypeStr=boolean  SampleTime=2e-08
  bits_per_subcarrier : Inport  Port=3  OutDataTypeStr=fixdt(0, 4, 0)  SampleTime=2e-08
  Bit Slice : hdlsllib/Logic and Bit Operations/Bit Slice  lidx=0  ridx=0
  Bit Slice1 : hdlsllib/Logic and Bit Operations/Bit Slice  lidx=1  ridx=0
  Bit Slice2 : hdlsllib/Logic and Bit Operations/Bit Slice  lidx=3  ridx=0
  Bit Slice3 : hdlsllib/Logic and Bit Operations/Bit Slice  lidx=5  ridx=0
  Constant{1..8} (8 alike) : Constant  Value=0  OutDataTypeStr=fixdt(1, 16, 14)  SampleTime=-1  LockScale=on
  Delay : Delay  DelayLength=1  InitialCondition=0  UseCircularBuffer=on
  Delay1 : Delay  DelayLength=1  InitialCondition=0  UseCircularBuffer=on
  Multiport Switch : MultiPortSwitch  DataPortOrder=Zero-based contiguous  Inputs=8  zeroidx=on  OutDataTypeStr=fixdt(1, 16, 14)  SaturateOnIntegerOverflow=off
  Real-Imag to Complex{1..4} (4 alike) : RealImagToComplex
  batID 0 : commdigbbndam3/Rectangular QAM Modulator Baseband  M=2  InType=Integer  Enc=Gray  Mapping=[0:15]  PowType=Average Power  MinDist=2  AvgPow=1  PeakPow=1  Ph=0  outDtype=Fixed-point  outWordLen=16  outUDDataType=sfix(16)  outFracLenMode=User-defined  outFracLen=14  outDataTypeStr=fixdt(1,16,14)  outLastDataTypeStr=fixdt(1,16,14)
      settings: LibrarySourceBlock=|
      | commhdldigbbndam/Rectangular QAM
      | Modulator
      | Baseband
  batID 1 : commdigbbndam3/Rectangular QAM Modulator Baseband  M=4  InType=Integer  Enc=Gray  Mapping=[0:15]  PowType=Average Power  MinDist=2  AvgPow=1  PeakPow=1  Ph=0  outDtype=Fixed-point  outWordLen=16  outUDDataType=sfix(16)  outFracLenMode=User-defined  outFracLen=14  outDataTypeStr=fixdt(1,16,14)  outLastDataTypeStr=fixdt(1,16,14)
      settings: LibrarySourceBlock=|
      | commhdldigbbndam/Rectangular QAM
      | Modulator
      | Baseband
  batID 12 : commdigbbndam3/Rectangular QAM Modulator Baseband  M=64  InType=Integer  Enc=Gray  Mapping=[0:15]  PowType=Average Power  MinDist=2  AvgPow=1  PeakPow=1  Ph=0  outDtype=Fixed-point  outWordLen=16  outUDDataType=sfix(16)  outFracLenMode=User-defined  outFracLen=14  outDataTypeStr=fixdt(1,16,14)  outLastDataTypeStr=fixdt(1,16,14)
      settings: LibrarySourceBlock=|
      | commhdldigbbndam/Rectangular QAM
      | Modulator
      | Baseband
  batID 8 : commdigbbndam3/Rectangular QAM Modulator Baseband  M=16  InType=Integer  Enc=Gray  Mapping=[0:15]  PowType=Average Power  MinDist=2  AvgPow=1  PeakPow=1  Ph=0  outDtype=Fixed-point  outWordLen=16  outUDDataType=sfix(16)  outFracLenMode=User-defined  outFracLen=14  outDataTypeStr=fixdt(1,16,14)  outLastDataTypeStr=fixdt(1,16,14)
      settings: LibrarySourceBlock=|
      | commhdldigbbndam/Rectangular QAM
      | Modulator
      | Baseband
  data_out : Outport  SampleTime=2e-08  InitialOutput=0
  valid_out : Outport  Port=2  SampleTime=2e-08  InitialOutput=0
  wires:
  batID 8/1 -> Multiport Switch/6
  batID 12/1 -> Multiport Switch/8
  batID 1/1 -> Multiport Switch/4
  batID 0/1 -> Multiport Switch/3
  Real-Imag to Complex4/1 -> Multiport Switch/9
  Real-Imag to Complex3/1 -> Multiport Switch/7
  Real-Imag to Complex2/1 -> Multiport Switch/5
  Real-Imag to Complex1/1 -> Multiport Switch/2
  Multiport Switch/1 -> Delay/1
  Delay1/1 -> valid_out/1
  Delay/1 -> data_out/1
  Constant8/1 -> Real-Imag to Complex4/2
  Constant7/1 -> Real-Imag to Complex3/2
  Constant6/1 -> Real-Imag to Complex3/1
  Constant5/1 -> Real-Imag to Complex1/2
  Constant4/1 -> Real-Imag to Complex2/2
  Constant3/1 -> Real-Imag to Complex1/1
  Constant2/1 -> Real-Imag to Complex2/1
  Constant1/1 -> Real-Imag to Complex4/1
  Bit Slice3/1 -> batID 12/1
  Bit Slice2/1 -> batID 8/1
  Bit Slice1/1 -> batID 1/1
  Bit Slice/1 -> batID 0/1
  bits_per_subcarrier/1 -> Multiport Switch/1
  valid_in/1 -> Delay1/1
  data_in/1 -> Bit Slice/1, Bit Slice1/1, Bit Slice2/1, Bit Slice3/1

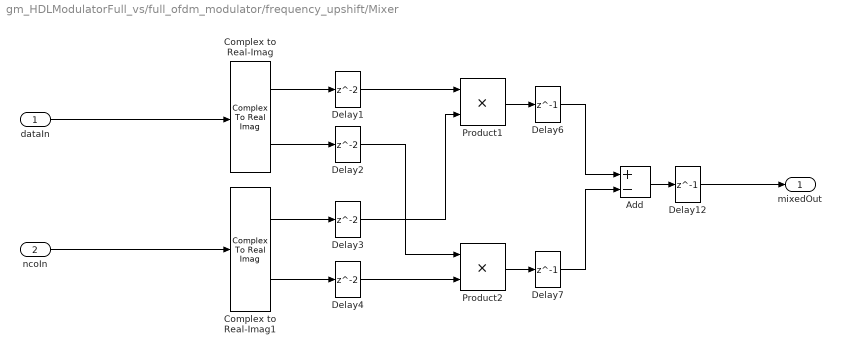
== system gm_HDLModulatorFull_vs/full_ofdm_modulator/frequency_upshift/Mixer ==
  dataIn : Inport  OutDataTypeStr=fixdt(1, 16, 14)  PortDimensions=1  SampleTime=1e-08
      settings: SignalType=complex
  ncoIn : Inport  Port=2  OutDataTypeStr=fixdt(1, 16, 14)  PortDimensions=1  SampleTime=1e-08
      settings: SignalType=complex
  Add : Sum  Inputs=+-  OutDataTypeStr=fixdt(1, 16, 14)  InputSameDT=on
  Complex to Real-Imag : ComplexToRealImag
  Complex to Real-Imag1 : ComplexToRealImag
  Delay{1..4} (4 alike) : Delay  InitialCondition=0
  Delay12 : Delay  DelayLength=1  InitialCondition=0
  Delay6 : Delay  DelayLength=1  InitialCondition=0
  Delay7 : Delay  DelayLength=1  InitialCondition=0
  Product1 : Product  OutDataTypeStr=fixdt(1, 16, 14)
  Product2 : Product  OutDataTypeStr=fixdt(1, 16, 14)
  mixedOut : Outport  SampleTime=1e-08
  wires:
  Product2/1 -> Delay7/1
  Product1/1 -> Delay6/1
  Delay7/1 -> Add/2
  Delay6/1 -> Add/1
  Delay4/1 -> Product2/2
  Delay3/1 -> Product1/2
  Delay2/1 -> Product2/1
  Delay12/1 -> mixedOut/1
  Delay1/1 -> Product1/1
  Complex to Real-Imag1/2 -> Delay4/1
  Complex to Real-Imag1/1 -> Delay3/1
  Complex to Real-Imag/2 -> Delay2/1
  Complex to Real-Imag/1 -> Delay1/1
  Add/1 -> Delay12/1
  ncoIn/1 -> Complex to Real-Imag1/1
  dataIn/1 -> Complex to Real-Imag/1

== system gm_HDLModulatorFull_vs/full_ofdm_modulator/interpolator/falling_edge_detector ==
  in : Inport  OutDataTypeStr=boolean  SampleTime=1e-08
  Delay : Delay  DelayLength=1  InitialCondition=0  UseCircularBuffer=on
  Logical Operator : Logic  IconShape=distinctive  AllPortsSameDT=off  OutDataTypeStr=boolean
  Logical Operator1 : Logic  Operator=NOT  IconShape=distinctive  AllPortsSameDT=off  OutDataTypeStr=boolean
  out : Outport  SampleTime=1e-08
  wires:
  Logical Operator1/1 -> Logical Operator/1
  Logical Operator/1 -> out/1
  Delay/1 -> Logical Operator/2
  in/1 -> Delay/1, Logical Operator1/1

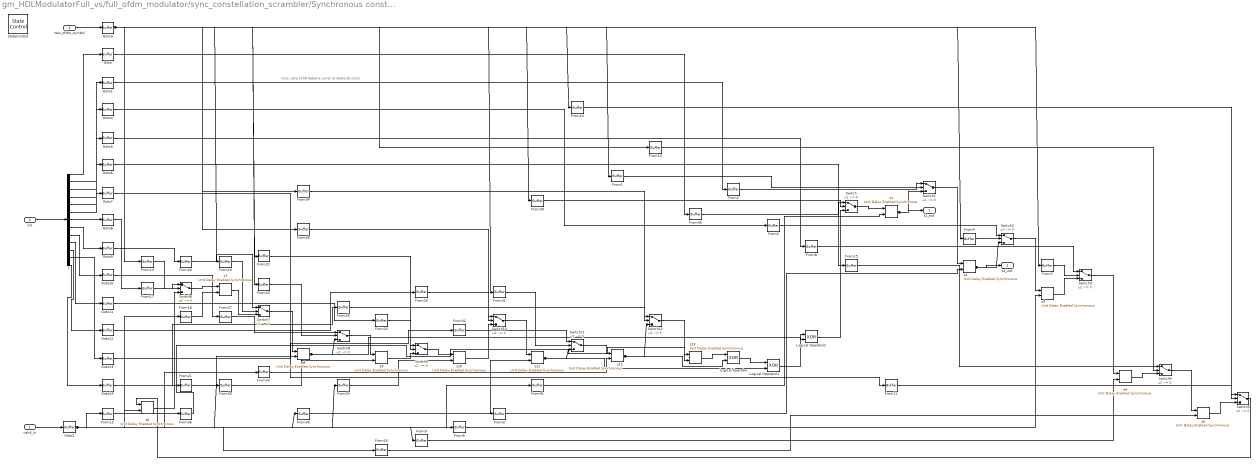
== system gm_HDLModulatorFull_vs/full_ofdm_modulator/sync_constellation_scrambler/Synchronous constellation scrambler ==
  note: nota: este LFSR deberia correr al doble de clock
  valid_in : Inport  OutDataTypeStr=boolean  PortDimensions=1  SampleTime=1e-08
  init : Inport  Port=2  OutDataTypeStr=boolean  PortDimensions=[1 13]  SampleTime=1e-08
  new_ofdm_symbol : Inport  Port=3  OutDataTypeStr=boolean  PortDimensions=1  SampleTime=1e-08
  From{1..36,39..41} (39 alike) : hdlmdlgenlib/Buffer
  Goto{,1..14} (15 alike) : hdlmdlgenlib/Buffer
  Logical Operator : Logic  Operator=XOR  AllPortsSameDT=off  OutDataTypeStr=boolean  SampleTime=1e-08
  Logical Operator1 : Logic  Operator=XOR  AllPortsSameDT=off  OutDataTypeStr=boolean  SampleTime=1e-08
  Logical Operator2 : Logic  Operator=XOR  AllPortsSameDT=off  OutDataTypeStr=boolean  SampleTime=1e-08
  StateControl : StateControl  StateControl=Synchronous
  Switch{,1..12} (13 alike) : Switch  Criteria=u2 ~= 0  Threshold=double(0)  OutDataTypeStr=boolean  SampleTime=1e-08  SaturateOnIntegerOverflow=off  InputSameDT=off
  s{1..13} (13 alike) : hdlsllib/Discrete/Unit Delay Enabled Synchronous  InitialCondition=double(0)  SampleTime=-1
  t : Demux  Outputs=13
  s1_out : Outport  SampleTime=1e-08  VectorParamsAs1DForOutWhenUnconnected=off
  s2_out : Outport  Port=2  SampleTime=1e-08  VectorParamsAs1DForOutWhenUnconnected=off
  wires:
  t/13 -> Goto14/1
  t/12 -> Goto13/1
  t/11 -> Goto12/1
  t/10 -> Goto11/1
  t/9 -> Goto10/1
  t/8 -> Goto9/1
  t/7 -> Goto8/1
  t/6 -> Goto7/1
  t/5 -> Goto6/1
  t/4 -> Goto5/1
  t/3 -> Goto4/1
  t/2 -> Goto1/1
  t/1 -> Goto/1
  Goto5/1 -> From8/1
  Goto4/1 -> From5/1
  Goto/1 -> From40/1
  Goto14/1 -> From35/1
  Goto13/1 -> From32/1
  Goto12/1 -> From29/1
  Goto10/1 -> From27/1
  Goto11/1 -> From23/1
  Goto9/1 -> From20/1
  Goto1/1 -> From2/1
  Goto8/1 -> From17/1
  Goto6/1 -> From15/1
  Goto2/1 -> From12/1, From16/1, From18/1, From21/1, From24/1, From28/1, From3/1, From30/1, From33/1, From36/1, From41/1, From6/1, From9/1
  Goto7/1 -> From11/1
  Goto3/1 -> From1/1, From10/1, From13/1, From14/1, From19/1, From22/1, From25/1, From26/1, From31/1, From34/1, From39/1, From4/1, From7/1
  s9/1 -> Switch9/3
  s8/1 -> Logical Operator2/2, Switch8/3
  s7/1 -> Switch7/3
  s6/1 -> Switch6/3
  s5/1 -> Switch5/3
  s4/1 -> Switch4/3
  s3/1 -> Switch3/3
  s2/1 -> s2_out/1, Switch2/3
  s13/1 -> Logical Operator/1
  s12/1 -> Logical Operator/2, Switch12/3
  s11/1 -> Logical Operator1/2, Switch11/3
  s10/1 -> Switch10/3
  s1/1 -> s1_out/1, Switch1/3
  Switch9/1 -> s10/1
  Switch8/1 -> s9/1
  Switch7/1 -> s8/1
  Switch6/1 -> s7/1
  Switch5/1 -> s6/1
  Switch4/1 -> s5/1
  Switch3/1 -> s4/1
  Switch2/1 -> s3/1
  Switch12/1 -> s13/1
  Switch11/1 -> s12/1
  Switch10/1 -> s11/1
  Switch1/1 -> s2/1
  Switch/1 -> s1/1
  Logical Operator2/1 -> Switch/3
  Logical Operator1/1 -> Logical Operator2/1
  Logical Operator/1 -> Logical Operator1/1
  From9/1 -> s4/2
  From8/1 -> Switch3/1
  From7/1 -> Switch3/2
  From6/1 -> s3/2
  From5/1 -> Switch2/1
  From41/1 -> s1/2
  From40/1 -> Switch/1
  From4/1 -> Switch2/2
  From39/1 -> Switch/2
  From36/1 -> s13/2
  From35/1 -> Switch12/1
  From34/1 -> Switch12/2
  From33/1 -> s12/2
  From32/1 -> Switch11/1
  From31/1 -> Switch11/2
  From30/1 -> s11/2
  From3/1 -> s2/2
  From29/1 -> Switch10/1
  From28/1 -> s9/2
  From27/1 -> Switch8/1
  From26/1 -> Switch10/2
  From25/1 -> Switch8/2
  From24/1 -> s10/2
  From23/1 -> Switch9/1
  From22/1 -> Switch9/2
  From21/1 -> s8/2
  From20/1 -> Switch7/1
  From2/1 -> Switch1/1
  From19/1 -> Switch7/2
  From18/1 -> s7/2
  From17/1 -> Switch6/1
  From16/1 -> s5/2
  From15/1 -> Switch4/1
  From14/1 -> Switch6/2
  From13/1 -> Switch4/2
  From12/1 -> s6/2
  From11/1 -> Switch5/1
  From10/1 -> Switch5/2
  From1/1 -> Switch1/2
  new_ofdm_symbol/1 -> Goto3/1
  init/1 -> t/1
  valid_in/1 -> Goto2/1

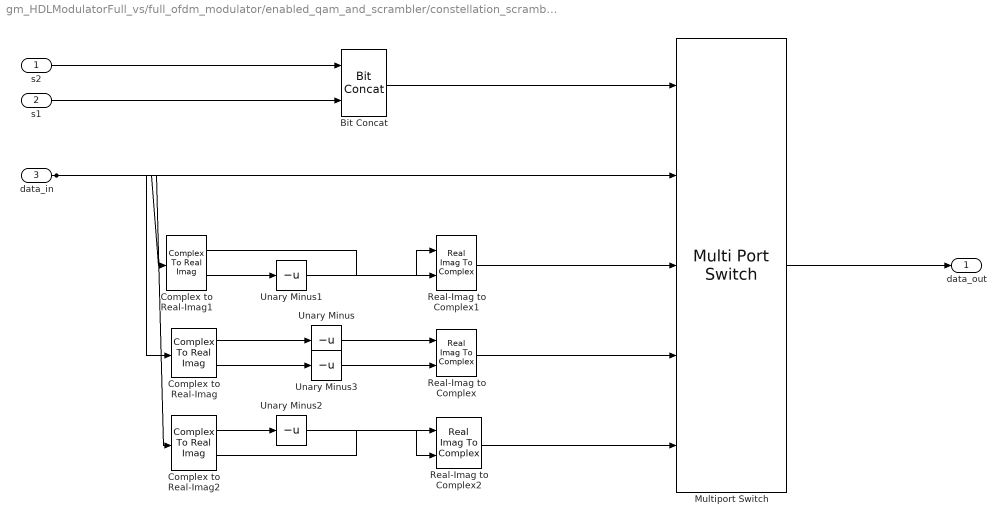
== system gm_HDLModulatorFull_vs/full_ofdm_modulator/enabled_qam_and_scrambler/constellation_scrambler/rotate ==
  s2 : Inport  OutDataTypeStr=boolean  PortDimensions=1  SampleTime=2e-08
  s1 : Inport  Port=2  OutDataTypeStr=boolean  PortDimensions=1  SampleTime=2e-08
  data_in : Inport  Port=3  OutDataTypeStr=fixdt(1, 16, 14)  PortDimensions=1  SampleTime=2e-08
      settings: SignalType=complex
  Bit Concat : hdlsllib/Logic and Bit Operations/Bit Concat  numInputs=2
  Complex to Real-Imag : ComplexToRealImag
  Complex to Real-Imag1 : ComplexToRealImag
  Complex to Real-Imag2 : ComplexToRealImag
  Multiport Switch : MultiPortSwitch  DataPortOrder=Zero-based contiguous  Inputs=4  zeroidx=on  OutDataTypeStr=fixdt(1, 16, 14)  SaturateOnIntegerOverflow=off  InputSameDT=off
  Real-Imag to Complex : RealImagToComplex
  Real-Imag to Complex1 : RealImagToComplex
  Real-Imag to Complex2 : RealImagToComplex
  Unary Minus{,1..3} (4 alike) : UnaryMinus
  data_out : Outport  SampleTime=2e-08  InitialOutput=0
  wires:
  Unary Minus3/1 -> Real-Imag to Complex/2
  Unary Minus2/1 -> Real-Imag to Complex2/2
  Unary Minus1/1 -> Real-Imag to Complex1/1
  Unary Minus/1 -> Real-Imag to Complex/1
  Real-Imag to Complex2/1 -> Multiport Switch/5
  Real-Imag to Complex1/1 -> Multiport Switch/3
  Real-Imag to Complex/1 -> Multiport Switch/4
  Multiport Switch/1 -> data_out/1
  Complex to Real-Imag2/2 -> Real-Imag to Complex2/1
  Complex to Real-Imag2/1 -> Unary Minus2/1
  Complex to Real-Imag1/2 -> Unary Minus1/1
  Complex to Real-Imag1/1 -> Real-Imag to Complex1/2
  Complex to Real-Imag/2 -> Unary Minus3/1
  Complex to Real-Imag/1 -> Unary Minus/1
  Bit Concat/1 -> Multiport Switch/1
  data_in/1 -> Complex to Real-Imag/1, Complex to Real-Imag1/1, Complex to Real-Imag2/1, Multiport Switch/2
  s1/1 -> Bit Concat/2
  s2/1 -> Bit Concat/1
